simulink model "x_vanderpol"  (Simulink 7.5)
settings: Solver=ode4  SolverMode=SingleTasking  StartTime=0.0  StopTime=5000  FixedStep=0.1  RelTol=1e-3  AbsTol=1e-6
libraries: simulink x3
Description:
  | The van der Pol Equation
  | 
  | This is a simulation of a nonlinear second order system.
settings Model: Creator=The MathWorks Inc.  LastModifiedBy=Dell  ExtModeAutoUpdateStatusClock=off
settings DataIOCC: ExternalInput=[]  InitialState=[]  LimitDataPoints=off  SaveOutput=off  SaveTime=off
settings OptimizationCC: BlockReduction=off  BooleanDataType=off  InlineInvariantSignals=on  InitFltsAndDblsToZero=on  BufferReusableBoundary=off
settings DebuggingCC: SaveWithParameterizedLinksMsg=none  SignalResolutionControl=TryResolveAllWithWarning  SolverPrmCheckMsg=none  MultiTaskDSMMsg=warning  MultiTaskCondExecSysMsg=none  BusObjectLabelMismatch=none  StrictBusMsg=None
settings HardwareCC: TargetUnknown=on
settings RTWCC: IncludeERTFirstTime=on
settings GRTTargetCC: TargetFcnLib=ansi_tfl_tmw.mat

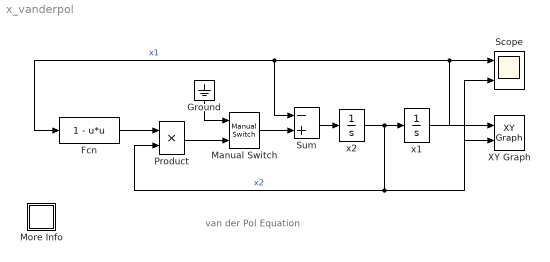
== system x_vanderpol ==
  note: van der Pol Equation
  Fcn : Fcn  Expr=1 - u*u
  Ground : Ground
  Manual Switch : simulink/Signal Routing/Manual Switch  SystemSampleTime=-1  sw=1  action=0  varsize=off
  More Info : Subsystem
      mask Display: disp('?')
  Product : Product  OutDataType=sfix(16)  OutScaling=2^0  SaturateOnIntegerOverflow=on  RndMeth=Zero  InputSameDT=on  OutDataTypeStr=Inherit: Same as first input
  Scope : Scope  NumInputPorts=2
      settings: TickLabels=on  TimeRange=50  YMin=-2.5~-3  YMax=2.5~3  DataFormat=Array
  Sum : Sum  Inputs=-+  OutDataType=sfix(16)  OutScaling=2^0  SaturateOnIntegerOverflow=on  InputSameDT=on  OutDataTypeStr=Inherit: Same as first input
  XY Graph : simulink/Sinks/XY Graph  SystemSampleTime=-1  xmin=-5  xmax=5  ymin=-5  ymax=5  st=-1
  x1 : Integrator  InitialCondition=-1
  x2 : Integrator  InitialCondition=3
  wires:
  Sum/1 -> x2/1
  x2/1 -> x1/1, Product/2, XY Graph/2, Scope/2  "x2"
  x1/1 -> Fcn/1, Sum/1, XY Graph/1, Scope/1  "x1"
  Fcn/1 -> Product/1
  Manual Switch/1 -> Sum/2
  Product/1 -> Manual Switch/2
  Ground/1 -> Manual Switch/1

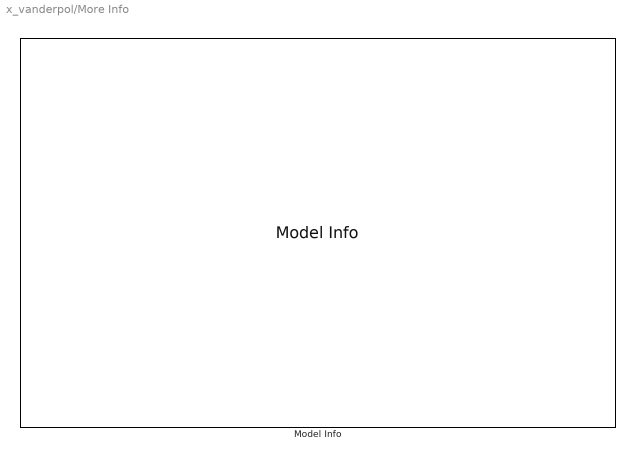
== system x_vanderpol/More Info ==
  Model Info : simulink/Model-Wide Utilities/Model Info  SystemSampleTime=-1  InitialBlockCM=none  BlockCM=None  Frame=on  DisplayStringWithTags=|  HorizontalTextAlignment=Left  LeftAlignmentValue=0.02  SourceBlockDiagram=x_vanderpol  TagMaxNumber=20
      | Model Description:
      | -------------------
      | 
      | %<Description>
